simulink model "signal"  (R2018a)
settings: Solver=FixedStepAuto  StartTime=0.0  StopTime=200  FixedStep=0.1  RelTol=1e-3
libraries: simulink x2
settings Model: Creator=Administrator  LastModifiedBy=Administrator

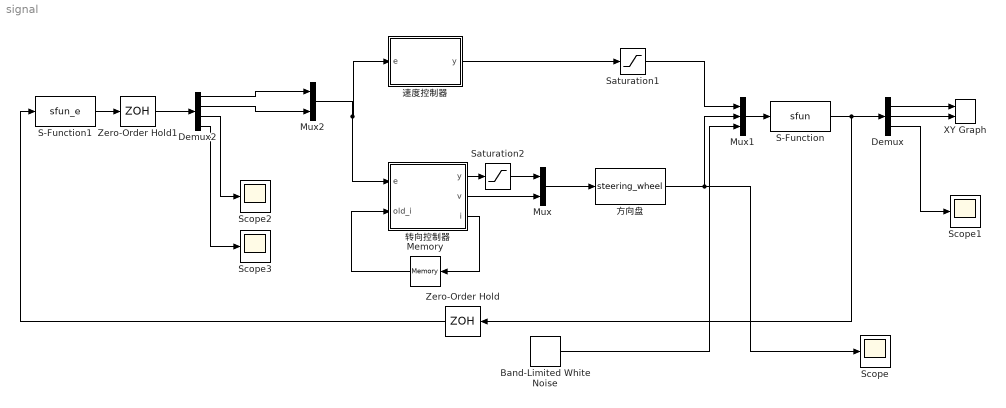
== system signal ==
  Band-Limited White Noise : simulink/Sources/Band-Limited White Noise  Cov=[0.00]  Ts=0.1  seed=[23341]
  Demux : Demux  Outputs=3
  Demux2 : Demux
  Memory : Memory
  Mux : Mux  Inputs=2
  Mux1 : Mux  Inputs=3
  Mux2 : Mux  Inputs=2
  S-Function : S-Function  FunctionName=sfun  SFunctionDeploymentMode=off  EnableBusSupport=off
  S-Function1 : S-Function  FunctionName=sfun_e  SFunctionDeploymentMode=off  EnableBusSupport=off
  Saturation1 : Saturate  UpperLimit=1  LowerLimit=0
  Saturation2 : Saturate  UpperLimit=pi/3  LowerLimit=-pi/3
  Scope{,1..3} (4 alike) : Scope
  XY Graph : simulink/Sinks/XY Graph  xmin=0  xmax=10  ymin=0  ymax=2  st=-1
  Zero-Order Hold : ZeroOrderHold  SampleTime=0.1
  Zero-Order Hold1 : ZeroOrderHold  SampleTime=-1
  方向盘 : S-Function  FunctionName=steering_wheel  SFunctionDeploymentMode=off  EnableBusSupport=off
  转向控制器 : MATLAB Function  TreatAsAtomicUnit=on
  速度控制器 : MATLAB Function  TreatAsAtomicUnit=on
  wires:
  S-Function/1 -> Zero-Order Hold/1, Demux/1
  S-Function1/1 -> Zero-Order Hold1/1
  Mux1/1 -> S-Function/1
  Demux/1 -> XY Graph/1
  Demux/2 -> XY Graph/2
  方向盘/1 -> Mux1/2, Scope/1
  速度控制器/1(y) -> Saturation1/1
  Saturation1/1 -> Mux1/1
  Demux/3 -> Scope1/1
  Band-Limited White Noise/1 -> Mux1/3
  转向控制器/3(i) -> Memory/1
  Memory/1 -> 转向控制器/2(old_i)
  Zero-Order Hold/1 -> S-Function1/1
  Saturation2/1 -> Mux/1
  转向控制器/2(v) -> Mux/2
  Mux/1 -> 方向盘/1
  转向控制器/1(y) -> Saturation2/1
  Zero-Order Hold1/1 -> Demux2/1
  Demux2/1 -> Mux2/1
  Demux2/2 -> Mux2/2
  Demux2/3 -> Scope2/1
  Demux2/4 -> Scope3/1
  Mux2/1 -> 转向控制器/1(e), 速度控制器/1(e)

== matlab function signal/转向控制器 ==
  data: e input; y output; v output; old_i input; i output
function [y, v, i] = fcn(e,old_i)
% y = atan(1.06 * cos(e(2))^3 * (3 * tan(e(2)) + 3 * e(1)));
i = old_i;
if e(1) < 0.15
    i = i + e(1);
end
if i > 200
    i = 200;
end
if i < -200
    i = -200;
end
y = e(2) + atan(1.2 * (e(1) + 1.06*sin(e(2))) / 1) ;
if y > 0
    v = 0.270526034059121;
else
    v = -0.270526034059121;
end

== matlab function signal/速度控制器 ==
  data: e input; y output
function y = fcn(e)

y = 0.7;
